simulink library "NCS_Library"  (R2019a)
settings: Solver=VariableStepAuto  StartTime=0.0  StopTime=10.0  RelTol=1e-3
values from neighbouring files (symbols this model uses):
  A = 10    [Parameter.m]
  band = 100000000    [Parameter.m]
  BER = 0    [Parameter.m]
  c = 5000000    [Parameter.m]
  c1 = 4.33    [Parameter.m]
  c2 = 3.16    [Parameter.m]
  CAN2EthernetDelay = 0.000    (= 0)    [Parameter.m]
  cR = 1.5*10^-3    (= 0.0015)    [Parameter.m]
  cw = (cwE * 2 + cwM * (nW_ges-2))/nW_ges    (= 0.1475)    [Parameter.m]
  cwE = 0.35    [Parameter.m]
  cwM = 0.08    [Parameter.m]
  Cycle_Controller = 0    [Parameter.m]
  CyclePLC = 24/1000    (= 0.024)    [Parameter.m]
  d = 800000    [Parameter.m]
  Dr = 0.92    [Parameter.m]
  Ethernet2CANDelay = 0.005    [Parameter.m]
  F_konst = 70892    [Parameter.m]
  FA = 100000    [Parameter.m]
  FB_WB_max = 10000    [Parameter.m]
  FBel_an = iG*nG*F_KZmax*nBan*R_mR/(Dr/2)    (= 28197.4297239)    [Parameter.m]
  FBel_frei = iG*nG*F_KZmax*nBfrei*R_mW/(Dr/2)    (= 29270.6882948)    [Parameter.m]
  Fmaxdyn = 300000    [Parameter.m]
  g = 9.81    [Parameter.m]
  i = 0    [Parameter.m]
  J = 1/2*mA*(Dr/2)^2    (= 158.7)    [Parameter.m]
  k1 = 0.095    [Parameter.m]
  k2 = 9.26/3.6    (= 2.57222222222)    [Parameter.m]
  k3 = 4.63/3.6    (= 1.28611111111)    [Parameter.m]
  mges = 58000    [Parameter.m]
  mu = [mu1 mu2]    [Parameter.m]
  muBel1 = 0.42    [Parameter.m]
  muBel2 = 0.36    [Parameter.m]
  n = 0.001    [Parameter.m]
  n_Mg = 4    [Parameter.m]
  n_WB = 4    [Parameter.m]
  nA = 4    [Parameter.m]
  nBan = 2    [Parameter.m]
  nBfrei = 3    [Parameter.m]
  nM = 4    [Parameter.m]
  nW_an = 4    [Parameter.m]
  P_max = 8200000    [Parameter.m]
  Q = 10    [Parameter.m]
  r_reib = 600    [Parameter.m]
  rho = 1.08    [Parameter.m]
  rhoL = 1.225    [Parameter.m]
  Size = 8    [Parameter.m]
  slip = [s1 s2]    [Parameter.m]
  tol = 0.05    [Parameter.m]
  v00 = 100/3.6    (= 27.7777777778)    [Parameter.m]
  v_grenz = 60/3.6    (= 16.6666666667)    [Parameter.m]
  v_opt = 75/3.6    (= 20.8333333333)    [Parameter.m]
  W_opt = 0.5    [Parameter.m]
  WB = 1    [Parameter.m]
  y_opt = sqrt(W_opt)/((1+sqrt(W_opt))^2+W_opt)    [Parameter.m]
undefined symbols (not defined in the file or in its folder): BUSCapacity, CableLength, controlGate, D_dyn, D_mg, EnableBurst, EnableToF, entity, Entity_out, Gate, Gate_4, Gate_5, Gate_ACK, Gate_copy, Gate_RX, getData, gettime, I_dyn, I_mg, m, magnitude, P_dyn, P_mg, ReadAttributes, readdata, ReadData, ReadSize, sigbuilder_block, Timeout, ToB, ToF, v0, v_d, v_soll
libraries: simulink x176, $bdroot x102
(part 12 of 12)

== stateflow chart NCS_Library/Network/CAN/CAN Node 2/Reception Control ==
  settings: enableNonTerminalStates=1
  state Process
    en:
    Port.data=S;
    send(Port);
  state [Status,Ack] = Compute(rx_id,loss,rx_rtr,rx_data,tx_id,tx_rtr,tx_data) [function]
  (default) -> Process : {S=1; Ack=0; TX_ID=-1; TX_RTR=0; TX_Data=0;}
  Process -> Process [order 1] : TX{TX_ID=TX.data.ID; TX_RTR=TX.data.RTR; TX_Data=TX.data.Data;}
  (junction 12) -> Process [order 1] : [Ack==1]{Success.data=1; send(Success);}
  (junction 12) -> Process [order 2] : [Ack==0]{ReTX.data=1; send(ReTX);}
  Process -> (junction 12) [order 2] : RX{[S,Ack]=Compute(RX.data.ID,...
      |                         RX.data.RndLoss, ...
      |                         RX.data.RTR, ...
      |                         RX.data.Data, ...
      |                         TX_ID, ...
      |                         TX_RTR, ...
      |                         TX_Data);}
  data: Status function_output; Ack function_output; rx_id function_input double size=1; loss function_input double size=1; rx_rtr function_input double size=1; rx_data function_input double size=1; tx_id function_input double size=1; tx_rtr function_input double size=1; tx_data function_input double size=1; TX input Bus: CAN_Message; RX input Bus: CAN_Message; S local; Ack local; TX_ID local; TX_RTR local; TX_Data local; Port output; Success output; ReTX output

== matlab function NCS_Library/Network/CAN/CAN Node 2/Reception Control/Compute/MATLAB Function ==
  data: ID0 input; ACK output; RTR0 input; Data0 input; ID1 input; RTR1 input; Data1 input; Loss input
function ACK = fcn(ID0,RTR0,Data0,ID1,RTR1,Data1,Loss)
% Compare the message ID, RTR, Data fields to acknowledge a successful send

if (ID0 == ID1 && RTR0 == RTR1 && Data0 == Data1 && Loss < 1)
    ACK = 1;
else
    ACK = 0;
end

== stateflow chart NCS_Library/Network/Applications/Watch Dog/Timeout Watch Dog ==
  state Init
    en: Failed = 0;
    en: Time=0;
    du: Time=GetTime;
  state Device_OK
    en: Time=0;
  state Wait
    en: LstTime = GetTime;
    du: Time=GetTime;
  state Time = GetTime [function]
  state Device_Failed
    en: Failed = 1;
  (default) -> Init
  Init -> Device_OK : [Time > 5]
  Wait -> Device_OK [order 2] : [Msg==1]
  Device_OK -> Wait
  Wait -> Device_Failed [order 1] : [Time - LstTime > Timeout]
  data: Time function_output; Failed output; Msg input; LstTime local; Time local; Timeout input

== matlab function NCS_Library/Network/Applications/Multiplexer/Mux U ==
  data: U input; U_out output
function U_out = MuxU(U)

U_out = [U(:,2), U(:,2), U(:,2), U(:,2)];

== matlab function NCS_Library/Network/Applications/NetworkSelector/Demux CAN ==
  data: U input; u1 output; u2 output; u3 output; u4 output
function [ u1, u2, u3, u4 ] = DemuxCAN(U)

u1 = U(:,1);
u2 = U(:,2);
u3 = U(:,3);
u4 = U(:,4);

== matlab function NCS_Library/Network/Applications/NetworkSelector/Demux CAN1 ==
  data: U input; u1 output; u2 output; u3 output; u4 output
function [ u1, u2, u3, u4 ] = DemuxCAN(U)

u1 = U(:,1);
u2 = U(:,2);
u3 = U(:,3);
u4 = U(:,4);

== matlab function NCS_Library/Network/ETB/Controller Interface/Subsystem/Mux Y_M ==
  data: in1 input; Y_M output; in2 input; in3 input; in4 input
function Y_M = MuxY_M(in1,in2,in3,in4)

Header = [1;0;0];

Y_M = [Header, in1(:,2), in2(:,2), in3(:,2), in4(:,2), zeros(3,15)];

== matlab function NCS_Library/Network/Applications/Multiplexer/Mux Consist ==
  data: in_1 input; out output; in_2 input
function out = MuxConsist(in_1, in_2)

out = [in_1; in_2];

== matlab function NCS_Library/Network/Applications/Multiplexer/Demux Consist ==
  data: in input; out_1 output; out_2 output
function [out_1, out_2] = DemuxConsist(in)

out_1 = in(1:3,:);
out_2 = in(4:6,:);

== matlab function NCS_Library/Network/Applications/Multiplexer/MUX ECN ==
  data: in1 input; U output; in2 input; in3 input; in4 input
function U = MuxU(in1,in2,in3,in4)

U = zeros(3,4);
U(:,1) = in1(:,2);
U(:,2) = in2(:,2);
U(:,3) = in3(:,2);
U(:,4) = in4(:,2);

== matlab function NCS_Library/Network/Applications/Multiplexer/MuxCAN ==
  data: u1 input; U output; u2 input; u3 input; u4 input
function U = MuxCAN(u1,u2,u3,u4)

U = [u1, u2, u3, u4];

end

== stateflow chart NCS_Library/Network/Gateway/Gateway2/CAN Interface/CAN Interface/Reception Control ==
  settings: enableNonTerminalStates=1
  state Process
    en:
    Port.data=S;
    send(Port);
  state [Status,Ack] = Compute(rx_id,loss,rx_rtr,rx_data,tx_id,tx_rtr,tx_data) [function]
  (default) -> Process : {S=1; Ack=0; TX_ID=-1; TX_RTR=0; TX_Data=0;}
  Process -> Process [order 1] : TX{TX_ID=TX.data.ID; TX_RTR=TX.data.RTR; TX_Data=TX.data.Data;}
  (junction 12) -> Process [order 1] : [Ack==1]{Success.data=1; send(Success);}
  (junction 12) -> Process [order 2] : [Ack==0]{ReTX.data=1; send(ReTX);}
  Process -> (junction 12) [order 2] : RX{[S,Ack]=Compute(RX.data.ID,...
      |                         RX.data.RndLoss, ...
      |                         RX.data.RTR, ...
      |                         RX.data.Data, ...
      |                         TX_ID, ...
      |                         TX_RTR, ...
      |                         TX_Data);}
  data: Status function_output; Ack function_output; rx_id function_input double size=1; loss function_input double size=1; rx_rtr function_input double size=1; rx_data function_input double size=1; tx_id function_input double size=1; tx_rtr function_input double size=1; tx_data function_input double size=1; TX input Bus: CAN_Message; RX input Bus: CAN_Message; S local; Ack local; TX_ID local; TX_RTR local; TX_Data local; Port output; Success output; ReTX output

== matlab function NCS_Library/Network/Gateway/Gateway2/CAN Interface/CAN Interface/Reception Control/Compute/MATLAB Function ==
  data: ID0 input; ACK output; RTR0 input; Data0 input; ID1 input; RTR1 input; Data1 input; Loss input
function ACK = fcn(ID0,RTR0,Data0,ID1,RTR1,Data1,Loss)
% Compare the message ID, RTR, Data fields to acknowledge a successful send

if (ID0 == ID1 && RTR0 == RTR1 && Data0 == Data1 && Loss < 1)
    ACK = 1;
else
    ACK = 0;
end

== stateflow chart NCS_Library/Network/Gateway/Gateway2/CAN Interface/Save Data/Hold Data ==
  state Init
    en: SavedData=InData;
  state Save_Data
    du: OutData=SavedData;
  state Push_Data
    en: OutData=SavedData;
  (default) -> Init
  Init -> Save_Data
  Push_Data -> Save_Data
  Save_Data -> Push_Data : [Flush==1]{SavedData=InData;}
  data: Flush input; InData input; SavedData local; OutData output

== matlab function NCS_Library/Network/Gateway/Gateway2/CAN Interface/Save Data/MATLAB Function ==
  data: refresh input; write input; Type input; Data input; M_Data output; M_Data_old input
function M_Data = SaveData (refresh, write, Type, Data, M_Data_old)
%% Init
M_Data = zeros(3,20);
M_Data(1,1) = 1;

if refresh
    % refresh matrix
else
    % save data in matrix
    M_Data = M_Data_old;
    if write && Type > 0 && Type < 3
        if M_Data(1,1) == 1
            % no data saved yet
            M_Data(Type,2) = Data;          % save data
            M_Data(1,1) = M_Data(1,1)+1;    % update length
        else
            % compare the data to write with the data already saved in the matrix
            for i=2:M_Data(1,1)+1
                if M_Data(1,i) ~= 0 || M_Data(2,i) ~= 0 || M_Data(3,i) ~= 0
                    % there is data at current position
                    if M_Data(Type,i) == Data
                        % data on current position is data to write
                        break;  % data already saved in Ethernet entity
                    end
                else
                    M_Data(Type,i) = Data;          % save data
                    M_Data(1,1) = M_Data(1,1)+1;    % update length
                    break;  % finished
                end
            end % endfor
        end
    end %endif write
end % endif refresh
end % function

== matlab function NCS_Library/Network/Gateway/Gateway2/Ethernet Interface/Buffer ==
  data: updatedBuffer input; Push input; Buffer output; Data input; data output
function [Buffer, data] = GatewayBuffer(updatedBuffer, Push, Data)

%% Init
Buffer = zeros(3,100);
FIN = 0;

Buffer = updatedBuffer;
%% Write to buffer
for i=2:Data(1,1)
    for j=1:length(Buffer)
        if Buffer(1,j) == 0 && Buffer(2,j) == 0 && Buffer(3,j) == 0
            % free position
            % save data
            Buffer(:,j) = Data(:,i);
            break;

        elseif Data(1,i) == Buffer(1,j) && Data(2,i) == Buffer(2,j) && Data(3,i) == Buffer(3,j)
            % data already in buffer
            FIN = 1;
            break;
        end
    end % end for
    
    if FIN
        % data already in buffer
        break;
    end
end % end for

%% Push
if Push
    % Read from buffer
    data = Buffer(:,1);

    % Udpdate buffer
    Buffer(:,1:length(Buffer)-1) = Buffer(:,2:length(Buffer));
else
    data = [0;0;0];
end

end % end function

== matlab function NCS_Library/Network/Gateway/Gateway2/Ethernet Interface/MATLAB Function ==
  data: u input; msgType output
function msgType = GetmsgType(u)

switch u
    case 1
        msgType = 11;
    case 2
        msgType = 13;
    case 3
        msgType = 13;
    otherwise
        msgType = 0;
end
end % end function

== matlab function NCS_Library/Network/Gateway/Gateway2/Ethernet Interface/MATLAB Function1 ==
  data: u input; y output
function y = fcn(u)

m = length(u);
ADD = zeros(m,2);
y = [u ADD];

== matlab function NCS_Library/Network/Applications/Multiplexer/Mux Reference Y_M ==
  data: in1 input; Y_M output; in2 input; in3 input; in4 input
function Y_M = MuxY_M(in1,in2,in3,in4)

Header = [1;0;0];
Y_M = [Header, in1, in2, in3, in4, zeros(3,15)];

== matlab function NCS_Library/Network/Gateway/Gateway2/Ethernet Interface/Subsystem4/MATLAB Function ==
  data: Data input; NEW output; Change input
function NEW = DetectNewData(Data, Change)

NEW = 0;
changed = 0;
for i=1:3
    for j=1:20
        if Change(i,j) ~= 0
            changed = 1;
            break;
        end
    end
end
        
if changed
    if Data(1,1) < 2
        % Data is empty
        NEW = 0;
    else
        % New Data
        NEW = Data(1,1)-1;
    end
end

end

== matlab function NCS_Library/Network/Applications/Multiplexer/Mux ==
  data: in_Y_M input; in_U input; out output
function out = Mux(in_Y_M,in_U)

out = [ in_Y_M, in_U ];

== matlab function NCS_Library/Network/Applications/Multiplexer/Mux y_m ==
  data: y_M input; Data output
function Data = MuxData(y_M)
% Save sensor signal (1x1) in valid data matrix (3x20)
Data = zeros(3,20);
Data(1,1) = 2;
Data(:,2) = y_M;

== matlab function NCS_Library/Network/Applications/NetworkSelector/Demux ==
  data: in input; U output; Y_M output
function [U, Y_M ] = Demux(in)

U = in(:,21:24);
Y_M = in(:,1:20);

== matlab function NCS_Library/Network/Applications/NetworkSelector/Demux Consist ==
  data: in input; out_1 output; out_2 output
function [out_1, out_2] = DemuxConsist(in)

out_1 = in(1:3,:);
out_2 = in(4:6,:);

== matlab function NCS_Library/Network/Applications/NetworkSelector/Demux1 ==
  data: in input; U output; Y_M output
function [U, Y_M ] = Demux(in)

U = in(:,21:24);
Y_M = in(:,1:20);
